simulink model "ctrl_student_HILWorksForCaseD"  (R2015a)
settings: Solver=ode3  StartTime=0.0  StopTime=inf  FixedStep=0.01  RelTol=1e-3
values from neighbouring files (symbols this model uses):
  DesiredPath = 0    [Innput.m]    (also in Input_v3.m = 1)
  Elipscenter_radi = [6 5;0 3 ]    [Innput.m]    (also in Input_v3.m)
  K = [2;10]    [Input_v3.m]
  K1 = diag([1,1,4])    [Input_v3.m]
  K2 = diag([200,50,3])    [Input_v3.m]    (also in inputDPgains.m = [1 0 0; 0 1 0; 0 0 1])
  l1 = [1 0 0;0 1 0;0 0 0.05]    [Input_v3.m]    (also in inputDPgains.m = [1 0 0; 0 1 0; 0 0 1])
  l2 = [1 0 0;0 1 0;0 0 0.05]    [Input_v3.m]    (also in inputDPgains.m = [1 0 0; 0 1 0; 0 0 1])
  l3 = [1 0 0;0 1 0;0 0 0.05]    [Input_v3.m]    (also in inputDPgains.m = [1 0 0; 0 1 0; 0 0 1])
  LAW = 1    [Innput.m]    (also in Input_v3.m = 0)
  lim = [1.00;-20;6.45/2;-6.45/2]    [Innput.m]    (also in Input_v3.m = [20;-20;9;-9])
  lim_2 = [1.5;-22;7;-7]    [Innput.m]    (also in Input_v3.m = [25;-25;10;-10])
  m = 14.79    [Input_v3.m]    (also in ctrl_student_init.m)
  mu = mu(1)    [Innput.m]    (also in Input_v3.m = 0.001)
  pd = [2 10;0 4]    [Input_v3.m]
  T_initialDP = T_initialDP*100    (= 6000)    [Input_v3.m]
  U_ref = 0.1    [Innput.m]    (also in Input_v3.m)
libraries: dspstat3 x1, simulink x1
(part 4 of 4)

== matlab function ctrl_student_HILWorksForCaseD/ControllerAndParanetrization/Controller1/Controller/Controller/MATLAB Function1 ==
  data: m input; M output
function M = fcn(m)
%% MATRICES

   I_z  =  1.7600;   x_g = 0.0375;       % x_g  =  0.0460; % Table B.1


%% Added mass
X_ud  =     -2.0;											% Table B.1
					Y_vd =     -1.0;	N_vd =    -0.0;		% Table B.1 guestimate
					Y_rd =      -0.0;	N_rd =    -1.0;		% Table B.1

%% Total mass matrix
m_11 = m-X_ud;
m_22 = m-Y_vd;
m_23 = m*x_g-Y_rd;
m_32 = m*x_g-N_vd;
m_33 = I_z-N_rd;

M    = [m_11 0    0
        0    m_22 m_23
        0    m_32 m_33];
end

== matlab function ctrl_student_HILWorksForCaseD/ControllerAndParanetrization/Controller1/Controller/Controller/alpha_1dott/MATLAB Function ==
  data: K_1 input; alpha_1dott output; nu input; r input; eta_ds input; R_T input; U_s input; s_dot input; eta_dss input; U_ss input; z_1 input
function alpha_1dott = fcn(K_1,nu,r,eta_ds,R_T,U_s,s_dot,eta_dss,U_ss,z_1)
%% term 1
S_T=[0 r 0;-r 0 0;0 0 0];

term1=S_T*R_T*eta_ds*U_s;
%% term 2

term2=K_1*(-S_T*z_1-nu);
%% term 3

term3=K_1*R_T*eta_ds*s_dot;
%% term 4

term4=R_T*eta_dss*s_dot*U_s;
%% term 5 

term5=R_T*eta_ds*U_ss*s_dot;
%% summary

alpha_1dott=term1+term2+term3+term4+term5;
end

== matlab function ctrl_student_HILWorksForCaseD/ThrustAllocationAndSaturation/actForces ==
  data: actSig input; tauAct output; satForces input
function tauAct  = act2Force(actSig,satForces)

t1=actSig(1)*satForces(1)*cos(actSig(2));
t2=actSig(3)*satForces(2)+actSig(1)*satForces(1)*sin(actSig(2));
t3=actSig(3)*satForces(2)*0.3875-actSig(1)*satForces(1)*sin(actSig(2))*0.4575;

tauAct=[t1;t2;t3];
end

== matlab function ctrl_student_HILWorksForCaseD/ThrustAllocationAndSaturation/Force Allocation ==
  data: current_mode input; tau_surge input; f_vspx output; tau_sway input; tau_yaw input; f_vspy output; f_bt output
function [f_vspx,f_vspy,f_bt] = fcn(current_mode,tau_surge,tau_sway,tau_yaw)
l_bt=0.3875;
l_vsp=-0.4575;

if current_mode==2
    f_vspx=tau_surge;
    f_vspy=0;
    f_bt=tau_yaw;
else
    %new equations from Silas 31/1/2017, based on Matlab inversion of B matrix
    f_vspx=tau_surge;
    f_vspy=(l_bt*tau_sway)/(l_bt - l_vsp) - tau_yaw/(l_bt - l_vsp);
    f_bt=tau_yaw/(l_bt - l_vsp) - (l_vsp*tau_sway)/(l_bt - l_vsp);
end

%original equations from 30/1/2017
% f_vspx=tau_surge;
% f_vspy=(tau_yaw-tau_sway*l_bt)/(l_vsp-l_bt);
% f_bt=tau_sway-f_vspy;

%tau_yaw = f_vspy*l_vsp+f_bt*l_bt
%tau_sway=f_vspy+f_bt
%solve for f_bt and f_vspy




end

== matlab function ctrl_student_HILWorksForCaseD/ThrustAllocationAndSaturation/Force2Control ==
  data: f_vspx input; u_vsp output; f_vspy input; f_bt input; alpha output; u_bt output; sat_forces input; satFlag output
function [u_vsp,alpha,u_bt,satFlag] = fcn(f_vspx,f_vspy,f_bt,sat_forces)

u_vsp=sqrt(f_vspx^2+f_vspy^2)/sat_forces(1);
u_bt=f_bt/sat_forces(2);
alpha=atan2(f_vspy,f_vspx);

if abs(u_vsp) > 1
    sf=1/abs(u_vsp);
    satFlag=1;
elseif abs(u_bt) > 1
    sf=1/abs(u_bt);
    satFlag=1;
else
    sf=1;
    satFlag=0;
end

u_vsp=u_vsp*sf;
u_bt=u_bt*sf;

end

== matlab function ctrl_student_HILWorksForCaseD/safety zone /MATLAB Function1 ==
  data: R input; R_T output
function R_T = fcn(R)
R_T=transpose(R);
end

== matlab function ctrl_student_HILWorksForCaseD/ControllerAndParanetrization/Controller1/Control parameterization/BacksteppingParameterization /V_1s/Rotation Matrix ==
  data: yaw input; R output
function R = fcn(yaw)

R=[cos(yaw) -sin(yaw) 0;
    sin(yaw) cos(yaw) 0;
    0 0 1];

end

== matlab function ctrl_student_HILWorksForCaseD/ControllerAndParanetrization/Controller1/Control parameterization/BacksteppingParameterization /Z_1/R Transposed ==
  data: R input; R_T output
function R_T = fcn(R)

R_T=transpose(R);

end

== matlab function ctrl_student_HILWorksForCaseD/ControllerAndParanetrization/Controller1/Control parameterization/BacksteppingParameterization /Z_1/Rotation Matrix ==
  data: yaw input; R output
function R = fcn(yaw)

R=[cos(yaw) -sin(yaw) 0;
    sin(yaw) cos(yaw) 0;
    0 0 1];

end

== matlab function ctrl_student_HILWorksForCaseD/ControllerAndParanetrization/PathParameterization/PathGenerization_Ellips/Check_s/CheckS&getU ==
  data: s_inn input; s_out output; U output; U_ref input; Switch output
function [s_out,U,Switch]= fcn(s_inn,U_ref)

if s_inn>=1
    s_out=0;
    Switch=0;
else
    s_out=s_inn;
    Switch=1;
end

U=U_ref/2;%U scaled again for the ellipsoidal case

end

== matlab function ctrl_student_HILWorksForCaseD/ControllerAndParanetrization/PathParameterization/PathGenerization_Straight/Path parametization /Eta_ds/MATLAB Function ==
  data: x_d input; eta_ds_yaw output; y_d input; x_dd input; y_dd input
function eta_ds_yaw = fcn(x_d,y_d,x_dd,y_dd)

eta_ds_yaw=(x_d*y_dd-y_d*x_dd)/(y_d^2+x_d^2);

end

== matlab function ctrl_student_HILWorksForCaseD/ControllerAndParanetrization/PathParameterization/PathGenerization_Straight/Path parametization /Eta_ds/MATLAB Function1 ==
  data: x_d input; x_dd output; y_d input; s input; y_dd output; x_dPrev input; y_dPrev input; s_Prev input; s1 output
function [x_dd,y_dd,s1]= fcn(x_d,y_d,s,x_dPrev,y_dPrev,s_Prev)

Delta_x=x_d-x_dPrev;
Delta_y=y_d-y_dPrev;
Delta_s=s-s_Prev;


x_dd=Delta_x/Delta_s;
y_dd=Delta_y/Delta_s;

s1=s;

end

== matlab function ctrl_student_HILWorksForCaseD/ControllerAndParanetrization/PathParameterization/PathGenerization_Ellips/Path parametization /Subsystem/MATLAB Function ==
  data: Elipscenter_radi input; pd output; s input; pd_s output; eta_ds output; eta_dss output; U_ref input; U_ss output
function [pd,pd_s,eta_ds,eta_dss,U_ss] = fcn(Elipscenter_radi,s,U_ref)
pd=zeros(2,1);
pd_s=pd;
eta_ds=zeros(3,1);
eta_dss=zeros(3,1);

pd(1)=Elipscenter_radi(1,1)+cos(2*pi*s)*Elipscenter_radi(1,2);
pd(2)=Elipscenter_radi(2,1)+sin(2*pi*s)*Elipscenter_radi(2,2);

pd_s(1)=-2*pi*Elipscenter_radi(1,2)*sin(2*pi*s);
pd_s(2)=2*pi*Elipscenter_radi(2,2)*cos(2*pi*s);

eta_ds(1)=pd_s(1);
eta_ds(2)=pd_s(2);
x_dss=-4*pi^2*Elipscenter_radi(1,2)*cos(2*pi*s);
y_dss=-4*pi^2*Elipscenter_radi(2,2)*sin(2*pi*s);
x_ds=pd_s(1);
y_ds=pd_s(2);
eta_ds(3)=(x_ds*y_dss-x_dss*y_ds)/(x_ds^2+y_ds^2);
eta_dss(1)=x_dss;
eta_dss(2)=y_dss;

x_dsss=8*pi^3*Elipscenter_radi(1,2)*sin(2*pi*s);
y_dsss=-8*pi^3*Elipscenter_radi(2,2)*cos(2*pi*s);
term1=(x_ds*y_dsss-y_ds*x_dsss)/(x_ds^2+y_ds^2);
term2=-((x_ds*y_dss-y_ds*x_dss)*(2*x_ds*x_dss+2*y_ds*y_dss))/(x_ds^2+y_ds^2)^2;
eta_dss(3)=term1+term2;
U_ss=U_ref*(-x_ds*x_dss-y_ds*y_dss)/((x_ds^2+y_ds^2)^(1.5));
end

== matlab function ctrl_student_HILWorksForCaseD/ControllerAndParanetrization/PathParameterization/PathGenerization_Ellips/parameter generator/MATLAB Function1 ==
  data: SwitchSignal_In input; SwitchSignal_Out output
function SwitchSignal_Out = fcn(SwitchSignal_In)

if SwitchSignal_In==0
    SwitchSignal_Out=1;
else
    SwitchSignal_Out=0;
end
    
end

== matlab function ctrl_student_HILWorksForCaseD/ControllerAndParanetrization/PathParameterization/PathGenerization_Ellips/parameter generator/UpdateLaw ==
  data: s_dot output; p_d_sdot input; U_ref input; U_s output; V_1s input; mu input; eta_ds input; LAW input
function [s_dot,U_s ]= fcn(p_d_sdot,U_ref,V_1s,mu,eta_ds,LAW)


U_s=U_ref/(sqrt(p_d_sdot(1)^2+p_d_sdot(2)^2));
if LAW ==1

        s_dot=U_s-mu*V_1s;
else
        s_dot=U_s-mu/(sqrt(eta_ds(1)^2+eta_ds(2)^2))*V_1s;
end


end

== matlab function ctrl_student_HILWorksForCaseD/ControllerAndParanetrization/PathParameterization/PathGenerization_Straight/Path parametization /Subsystem/MATLAB Function ==
  data: InitPosOut output; DesPos input; s_in input; U_ref input; N_iteration input; N_in input; DesPosOut output; SwitchSignal_out output; N_out output; U output; s_out output; Start_time input; init_time output; flag output
function [InitPosOut,DesPosOut,SwitchSignal_out,N_out,U,s_out,init_time,flag]= fcn(DesPos,s_in,U_ref,N_iteration,N_in,Start_time)
[a,b]=size(DesPos);
N_max=b-1;
    init_time=zeros(2,1);
    init_time(1)=Start_time(1)+1;
    init_time(2)=Start_time(2);
   

    
    
if init_time(1)<N_iteration         % DP for N_iterations
    N_out=N_in;
    InitPosOut=DesPos(:,N_out);
    DesPosOut=DesPos(:,N_out+1);
    SwitchSignal_out=1;
    s_out=0;
    DP=1;
    flag=1;
    
else
    if N_in==N_max                  % if we are at final stretch
        if  s_in>=0.9999
            N_out=N_in;
            InitPosOut=DesPos(:,N_out);
            DesPosOut=DesPos(:,N_out+1);
            SwitchSignal_out=1;
            s_out=1;
            DP=1;
            flag=2;
            
        else
            N_out=N_in;
            InitPosOut=DesPos(:,N_in);
            DesPosOut=DesPos(:,N_in+1);
            SwitchSignal_out=1;
            s_out=s_in;
            DP=0;
            flag=3;
            
        end
    else
       if s_in>=0.9999
           if N_in+1 ==N_max
               SwitchSignal_out=0;
               flag=40;
           else
               SwitchSignal_out=0;
               flag=50;
           end
            N_out=N_in+1;
            InitPosOut=DesPos(:,N_out);
            DesPosOut=DesPos(:,N_out+1);
            s_out=1;
            DP=0;

       else 
            if init_time(2)==0;
                init_time(2)=1;
                SwitchSignal_out=0;
                flag=5.75;
            else
                SwitchSignal_out=1;
                flag=5.25;
            end
            N_out=N_in;
            InitPosOut=DesPos(:,N_in);
            DesPosOut=DesPos(:,N_in+1);
            s_out=s_in;
            DP=0;
            
        end
    end
    
end   
if DP==1
    U=0;
else
    U=U_ref*(1.01+ sin(2*pi*s_out-pi/2));
end

end

== matlab function ctrl_student_HILWorksForCaseD/ControllerAndParanetrization/PathParameterization/PathGenerization_Straight/parameter generator/MATLAB Function1 ==
  data: SwitchSignal_In input; SwitchSignal_Out output
function SwitchSignal_Out = fcn(SwitchSignal_In)

if SwitchSignal_In==0
    SwitchSignal_Out=1;
else
    SwitchSignal_Out=0;
end
    
end

== matlab function ctrl_student_HILWorksForCaseD/ControllerAndParanetrization/PathParameterization/PathGenerization_Straight/parameter generator/UpdateLaw ==
  data: s_dot output; p_d_sdot input; U_ref input; U_s output; V_1s input; mu input; eta_ds input; LAW input
function [s_dot,U_s ]= fcn(p_d_sdot,U_ref,V_1s,mu,eta_ds,LAW)


U_s=U_ref/(sqrt(p_d_sdot(1)^2+p_d_sdot(2)^2));
if LAW ==1

        s_dot=U_s-mu*V_1s;
else
        s_dot=U_s-mu/(sqrt(eta_ds(1)^2+eta_ds(2)^2))*V_1s;
end


end

== matlab function ctrl_student_HILWorksForCaseD/DPObserver1/Bias/bHatDot ==
  data: bHatDot output; L3 input; eta input; etaHat input
function bHatDot = fcn(L3,eta,etaHat)

bHatDot=L3*(eta-etaHat);
%bHatDot=[0;0;0];

end

== matlab function ctrl_student_HILWorksForCaseD/DPObserver1/D ==
  data: D output; etaHatDot input
function D = fcn(etaHatDot)

u=etaHatDot(1);     %u=0; 
v=etaHatDot(2);     %v=0; 
r=etaHatDot(3);     %r=0;

Xu=-0.6555;
Xuu=0.3545;
Xuuu=-3.787;
Yv=-1.33;
Yvv=-2.776;
Yvvv=-64.91;
Yr=-7.25;
Yrr=-3.45;
Yrrr=0;
Yrv=-0.805;
Yvr=-0.845;
Nv=0;
Nvv=-0.2088;
Nvvv=0;
Nr=-1.9;
Nrr=-0.75;
Nrrr=0;
Nrv=0.13;
Nvr=0.08;

d11=-Xu-Xuu*abs(u)-Xuuu*u^2;
d22=-Yv-Yvv*abs(v)-Yvvv*v^2-Yrv*abs(r);
d23=-Yr-Yvr*abs(v)-Yrr*abs(r)-Yrrr*r^2;
d32=-Nv-Nvv*abs(v)-Nvvv*v^2-Nrv*abs(r);
d33=-Nr-Nvr*abs(v)-Nrr*abs(r)-Nrrr*r^2;

D=[d11 0 0; 0 d22 d23; 0 d32 d33];

end

== matlab function ctrl_student_HILWorksForCaseD/DPObserver1/Subsystem/M ==
  data: M output
function M = void

m=14.79;
M=[m+2 0 0; 0 m+10 m*0.0375; 0 m*0.0375 1.76+1];

end

== matlab function ctrl_student_HILWorksForCaseD/DPObserver1/Subsystem/nuHatDot ==
  data: nuHat input; bHat input; D input; M input; L2 input; tau input; eta input; R input; etaHat input; nuHatDot output
function nuHatDot = fcn(nuHat,bHat,D,M,L2,tau,eta,R,etaHat)

%nuHatDot=inv(M)*(-D*nuHat+transpose(R)*bHat+tau+K2*transpose(R)*L2*(eta-etaHat));

nuHatDot=inv(M)*(-D*nuHat+transpose(R)*bHat+tau+transpose(R)*L2*(eta-etaHat));

end

== matlab function ctrl_student_HILWorksForCaseD/DPObserver1/calcR(psi)  ==
  data: psi input; R output
function R = fcn(psi)

R=[cos(psi) -sin(psi) 0; sin(psi) cos(psi) 0; 0 0 1];

end

== matlab function ctrl_student_HILWorksForCaseD/DPObserver1/etaHat/etaHatDot ==
  data: etaHat input; nuHat input; L1 input; eta input; R input; etaHatDot output
function etaHatDot = fcn(etaHat,nuHat,L1,eta,R)

%etaHatDot=zeros(3,1);
etaHatDot=R*nuHat+L1*(eta-etaHat);

end
